simulink model "swingup_nodamping"  (R2022b)
settings: Solver=VariableStepAuto  StartTime=0.0  StopTime=20  RelTol=1e-3
values from neighbouring files (symbols this model uses):
  g = 9.81    [startup.m]
  k = 1    [startup.m]
  L = 1    [startup.m]
  m = 1    [startup.m]
  theta0 = deg2rad(5)    [startup.m]
  theta_dot0 = 0    [startup.m]
libraries: simulink_extras x1
settings Model: Creator=logan  LastModifiedBy=logan

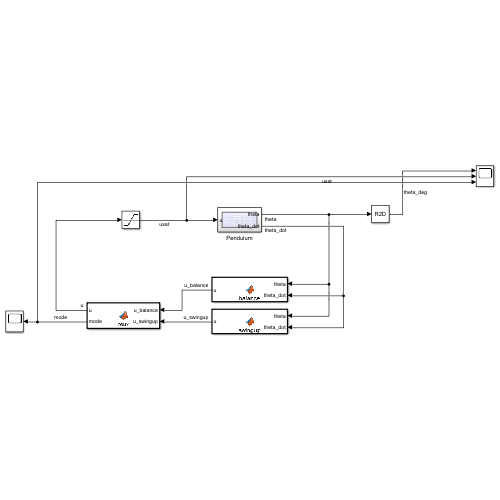
[thumbnail: Simulink's stored preview of the top-level diagram]
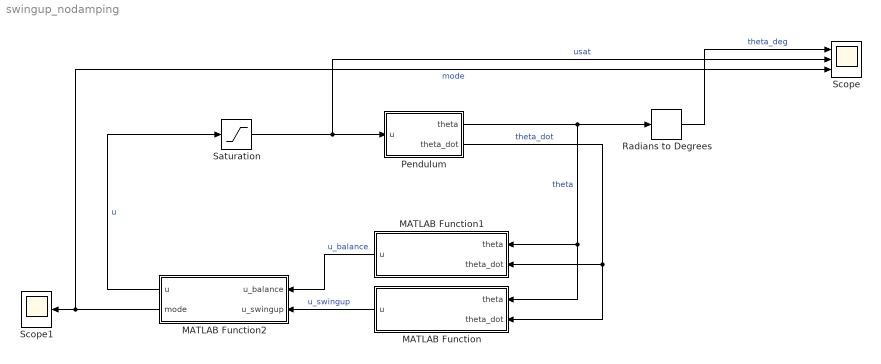
== system swingup_nodamping ==
  MATLAB Function : MATLAB Function  TreatAsAtomicUnit=on
  MATLAB Function1 : MATLAB Function  TreatAsAtomicUnit=on
  MATLAB Function2 : MATLAB Function  TreatAsAtomicUnit=on
  Pendulum : Subsystem
  Radians to Degrees : simulink_extras/Transformations/Radians to Degrees
  Saturation : Saturate  UpperLimit=1  LowerLimit=-1
  Scope : Scope  NumInputPorts=3
  Scope1 : Scope
  wires:
  Radians to Degrees/1 -> Scope/1  "theta_deg"
  Pendulum/1(theta) -> MATLAB Function/1(theta), MATLAB Function1/1(theta), Radians to Degrees/1  "theta"
  Pendulum/2(theta_dot) -> MATLAB Function/2(theta_dot), MATLAB Function1/2(theta_dot)  "theta_dot"
  Saturation/1 -> Scope/2, Pendulum/1(u)  "usat"
  MATLAB Function/1(u) -> MATLAB Function2/2(u_swingup)  "u_swingup"
  MATLAB Function1/1(u) -> MATLAB Function2/1(u_balance)  "u_balance"
  MATLAB Function2/1(u) -> Saturation/1  "u"
  MATLAB Function2/2(mode) -> Scope/3, Scope1/1  "mode"

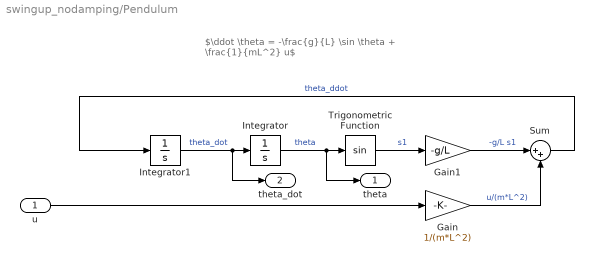
== system swingup_nodamping/Pendulum ==
  note: $\ddot \theta = -\frac{g}{L} \sin \theta + \frac{1}{mL^2} u$
  u : Inport
  Gain : Gain  Gain=1/(m*L^2)
  Gain1 : Gain  Gain=-g/L
  Integrator : Integrator  InitialCondition=theta0
  Integrator1 : Integrator  InitialCondition=theta_dot0
  Sum : Sum  Inputs=|++
  Trigonometric Function : Trigonometry
  theta : Outport
  theta_dot : Outport  Port=2
  wires:
  Integrator/1 -> theta/1, Trigonometric Function/1  "theta"
  Gain1/1 -> Sum/1  "-g/L s1"
  Trigonometric Function/1 -> Gain1/1  "s1"
  Integrator1/1 -> theta_dot/1, Integrator/1  "theta_dot"
  u/1 -> Gain/1
  Gain/1 -> Sum/2  "u/(m*L^2)"
  Sum/1 -> Integrator1/1  "theta_ddot"

== matlab function swingup_nodamping/MATLAB Function1 ==
  data: theta input; u output; theta_dot input; K parameter
function u = balance(theta, theta_dot, K)

% use LQR
theta_error = wrapTo2Pi(theta-pi);
u = -K*[theta_error; theta_dot];
% u = 12*theta_error;

== matlab function swingup_nodamping/MATLAB Function ==
  data: theta input; u output; theta_dot input; m parameter; L parameter; g parameter; k parameter
function u = swingup(theta, theta_dot, m, L, g, k)

E = 1/2*m*L^2*theta_dot^2 - m*g*L*cos(theta);
Ed = m*g*L;
E_tilde = E-Ed;

u = -k*theta_dot*E_tilde;

== matlab function swingup_nodamping/MATLAB Function2 ==
  data: u output; u_balance input; u_swingup input; mode output
function [u, mode] = mux(u_balance, u_swingup)

if abs(u_balance) < 1
    u = u_balance;
    mode = 1;
else
    u = u_swingup;
    mode = 0;
end
